simulink subsystem "suspension"  (R2024b)
settings: Solver=VariableStepAuto  StartTime=0.0  StopTime=10.0  RelTol=1e-3
model mask{ride_rate=0, damp_rate=0}
  mask prompts: ride_rate "Ride rate [N/m]"; damp_rate "Damping [N/(m/s)]"
settings Model: Creator=yevge  LastModifiedBy=yevge

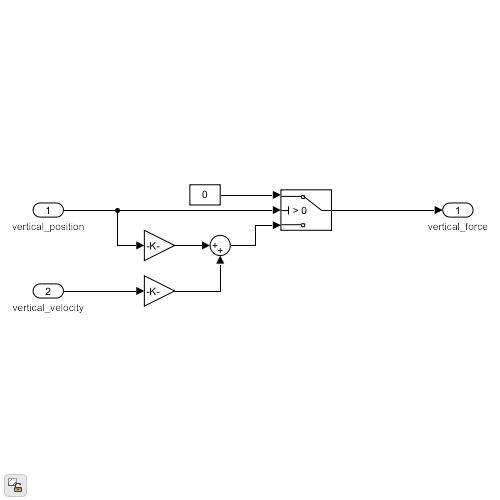
[thumbnail: Simulink's stored preview of the top-level diagram]
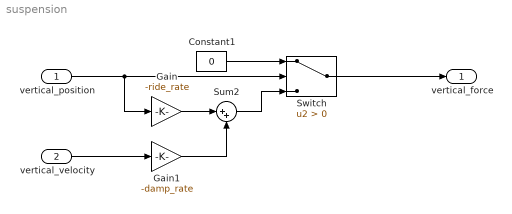
== system suspension ==
  vertical_position : Inport
  vertical_velocity : Inport  Port=2
  Constant1 : Constant  Value=0
  Gain : Gain  Gain=-ride_rate
  Gain1 : Gain  Gain=-damp_rate
  Sum2 : Sum  Inputs=|++
  Switch : Switch  Criteria=u2 > Threshold  SaturateOnIntegerOverflow=off  InputSameDT=off
  vertical_force : Outport
  wires:
  vertical_position/1 -> Switch/2, Gain/1
  Gain/1 -> Sum2/1
  vertical_velocity/1 -> Gain1/1
  Gain1/1 -> Sum2/2
  Sum2/1 -> Switch/3
  Constant1/1 -> Switch/1
  Switch/1 -> vertical_force/1
